simulink model "bondarko3Task"  (R2018a)
settings: Solver=VariableStepAuto  StartTime=0.0  StopTime=10.0  RelTol=1e-3
undefined symbols (not defined in the file): K, T
settings Model: Creator=Петр  LastModifiedBy=Петр

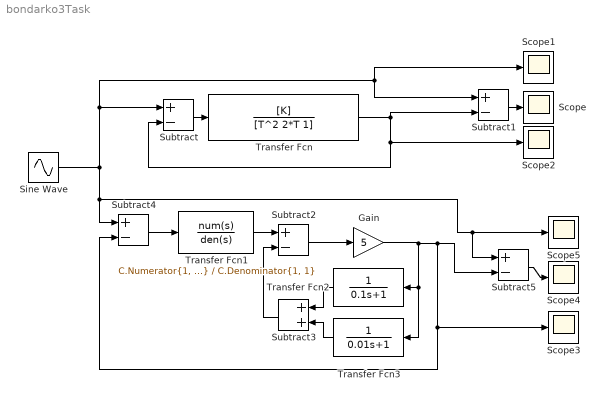
== system bondarko3Task ==
  Gain : Gain  Gain=5
  Scope{,1..5} (6 alike) : Scope
  Sine Wave : Sin  Frequency=3000  SampleTime=0
  Subtract{,1..2,4..5} (5 alike) : Sum  Inputs=+-
  Subtract3 : Sum
  Transfer Fcn : TransferFcn  Numerator=[K]  Denominator=[T^2 2*T 1]
  Transfer Fcn1 : TransferFcn  Numerator=C.Numerator{1, 1}  Denominator=C.Denominator{1, 1}
  Transfer Fcn2 : TransferFcn  Denominator=[0.1 1]
  Transfer Fcn3 : TransferFcn  Denominator=[0.01 1]
  wires:
  Subtract/1 -> Transfer Fcn/1
  Transfer Fcn/1 -> Subtract1/2, Subtract/2, Scope2/1
  Subtract1/1 -> Scope/1
  Sine Wave/1 -> Scope1/1, Subtract1/1, Subtract/1, Scope5/1, Subtract5/1, Subtract4/1
  Transfer Fcn1/1 -> Subtract2/1
  Subtract2/1 -> Gain/1
  Transfer Fcn2/1 -> Subtract3/1
  Transfer Fcn3/1 -> Subtract3/2
  Subtract3/1 -> Subtract2/2
  Subtract4/1 -> Transfer Fcn1/1
  Subtract5/1 -> Scope4/1
  Gain/1 -> Subtract5/2, Subtract4/2, Scope3/1, Transfer Fcn3/1, Transfer Fcn2/1
